simulink model "inprogress"  (R2017b)
settings: Solver=FixedStepAuto  StartTime=0.0  StopTime=10000  RelTol=1e-3  EnableMultiTasking=on
libraries: vexarmcortexlib x23
settings Model: ExtModeTrigDuration=25  Creator=Walt  LastModifiedBy=Walt
settings OptimizationCC: PassReuseOutputArgsAs=Individual arguments  MaxStackSize=64
settings DebuggingCC: ParameterTunabilityLossMsg=error
settings HardwareCC: ProdBitPerPointer=32  ProdBitPerSizeT=32  ProdBitPerPtrDiffT=32  ProdLargestAtomicInteger=Long  ProdLargestAtomicFloat=Double  ProdWordSize=32  ProdHWDeviceType=ARM Compatible->ARM Cortex
settings SFSimCC: MATLABDynamicMemAlloc=off
settings RTWCC: SystemTargetFile=ert.tlc  HardwareBoard=ARM Cortex-based VEX Microcontroller  TemplateMakefile=ert_default_tmf  GenerateReport=on  Toolchain=GNU Tools for VEX ARM Cortex  IncludeHyperlinkInReport=on  LaunchReport=on  GenerateTraceInfo=on  GenerateTraceReport=on  GenerateTraceReportSl=on  GenerateTraceReportSf=on  GenerateTraceReportEml=on
settings CodeAppCC: ForceParamTrailComments=on  IgnoreCustomStorageClasses=off  OperatorAnnotations=on  SimulinkDataObjDesc=on  SFDataObjDesc=on  InsertBlockDesc=on

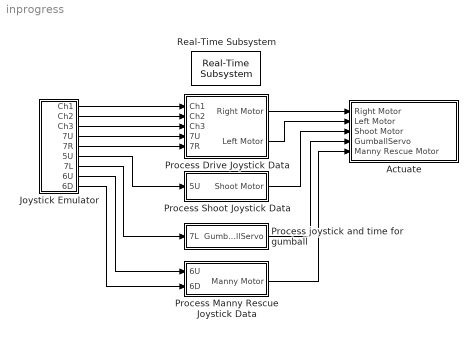
== system inprogress ==
  Actuate : Subsystem
  Joystick Emulator : Subsystem
  Process Drive Joystick Data : Subsystem
  Process Manny Rescue Joystick Data : Subsystem
  Process Shoot Joystick Data : Subsystem
  Process joystick and time for gumball : Subsystem
  Real-Time Subsystem : vexarmcortexlib/Utilities/Real-Time Subsystem  x=1
      settings: SourceProductName=Simulink Coder Support Package for ARM Cortex-based VEX Microcontroller  SourceProductBaseCode=EC_VEX_MICRO
  wires:
  Joystick Emulator/1(Ch1) -> Process Drive Joystick Data/1(Ch1)
  Joystick Emulator/2(Ch2) -> Process Drive Joystick Data/2(Ch2)
  Joystick Emulator/3(Ch3) -> Process Drive Joystick Data/3(Ch3)
  Joystick Emulator/5(7R) -> Process Drive Joystick Data/5(7R)
  Process Drive Joystick Data/1(Right Motor) -> Actuate/1(Right Motor)
  Process Drive Joystick Data/2(Left Motor) -> Actuate/2(Left Motor)
  Joystick Emulator/4(7U) -> Process Drive Joystick Data/4(7U)
  Joystick Emulator/6(5U) -> Process Shoot Joystick Data/1(5U)
  Process Shoot Joystick Data/1(Shoot Motor) -> Actuate/3(Shoot Motor)
  Joystick Emulator/8(6U) -> Process Manny Rescue Joystick Data/1(6U)
  Joystick Emulator/9(6D) -> Process Manny Rescue Joystick Data/2(6D)
  Process Manny Rescue Joystick Data/1(Manny Motor) -> Actuate/5(Manny Rescue Motor)
  Joystick Emulator/7(7L) -> Process joystick and time for gumball/1(7L)
  Process joystick and time for gumball/1(GumballServo) -> Actuate/4(GumballServo)

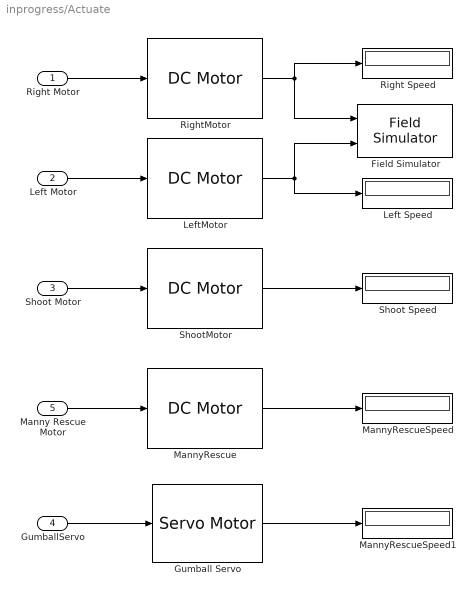
== system inprogress/Actuate ==
  Right Motor : Inport
  Left Motor : Inport  Port=2
  Shoot Motor : Inport  Port=3
  GumballServo : Inport  Port=4
  Manny Rescue Motor : Inport  Port=5
  Field Simulator : vexarmcortexlib/Utilities/Field Simulator  radius=4  space=8  range=200
      settings: SourceProductName=Simulink Coder Support Package for ARM Cortex-based VEX Microcontroller  SourceProductBaseCode=EC_VEX_MICRO
  Gumball Servo : vexarmcortexlib/Actuators/Servo Motor  motor=1  scaleFactor=60/127  SimulationOut=on
      settings: SourceProductName=Simulink Coder Support Package for ARM Cortex-based VEX Microcontroller  SourceProductBaseCode=EC_VEX_MICRO
  Left Speed : Display
  LeftMotor : vexarmcortexlib/Actuators/DC Motor  motor=2  scaleFactor=1/13.5  SimulationOut=on
      settings: SourceProductName=Simulink Coder Support Package for ARM Cortex-based VEX Microcontroller  SourceProductBaseCode=EC_VEX_MICRO
  MannyRescue : vexarmcortexlib/Actuators/DC Motor  motor=8  scaleFactor=1/13.5  SimulationOut=on
      settings: SourceProductName=Simulink Coder Support Package for ARM Cortex-based VEX Microcontroller  SourceProductBaseCode=EC_VEX_MICRO
  MannyRescueSpeed : Display
  MannyRescueSpeed1 : Display
  Right Speed : Display
  RightMotor : vexarmcortexlib/Actuators/DC Motor  motor=9  scaleFactor=1/13.5  SimulationOut=on
      settings: SourceProductName=Simulink Coder Support Package for ARM Cortex-based VEX Microcontroller  SourceProductBaseCode=EC_VEX_MICRO
  Shoot Speed : Display
  ShootMotor : vexarmcortexlib/Actuators/DC Motor  motor=3  scaleFactor=1/13.5  SimulationOut=on
      settings: SourceProductName=Simulink Coder Support Package for ARM Cortex-based VEX Microcontroller  SourceProductBaseCode=EC_VEX_MICRO
  wires:
  Shoot Motor/1 -> ShootMotor/1
  Manny Rescue Motor/1 -> MannyRescue/1
  Right Motor/1 -> RightMotor/1
  Left Motor/1 -> LeftMotor/1
  GumballServo/1 -> Gumball Servo/1
  RightMotor/1 -> Right Speed/1, Field Simulator/1
  LeftMotor/1 -> Field Simulator/2, Left Speed/1
  ShootMotor/1 -> Shoot Speed/1
  MannyRescue/1 -> MannyRescueSpeed/1
  Gumball Servo/1 -> MannyRescueSpeed1/1

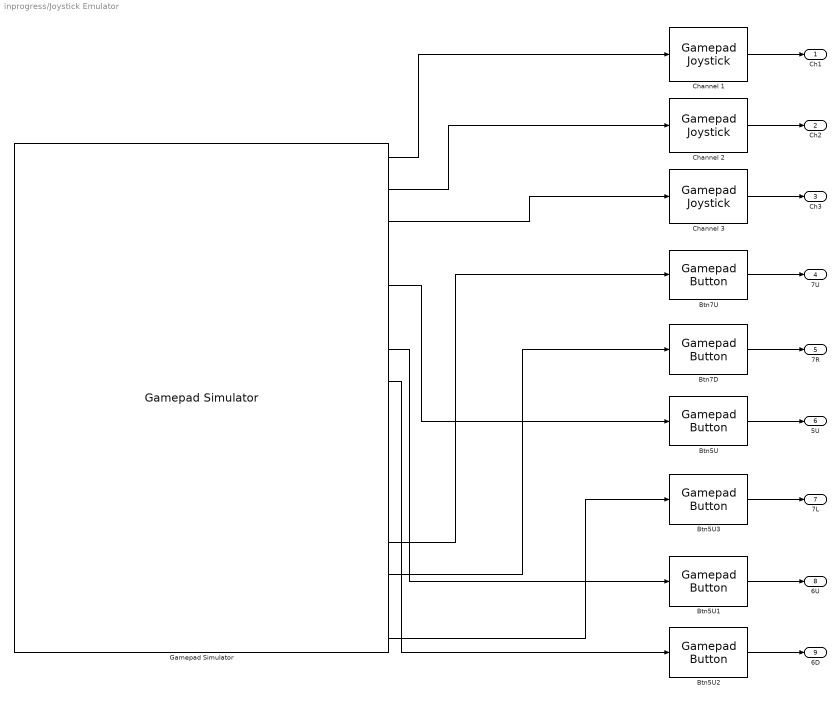
== system inprogress/Joystick Emulator ==
  Btn5U : vexarmcortexlib/Gamepad/Gamepad Button  joystick=1  chan=5  button56=Up  button78=Down  SimulationIn=on  SampleTime=0.2
      settings: SourceProductName=Simulink Coder Support Package for ARM Cortex-based VEX Microcontroller  SourceProductBaseCode=EC_VEX_MICRO
  Btn5U1 : vexarmcortexlib/Gamepad/Gamepad Button  joystick=1  chan=6  button56=Up  button78=Down  SimulationIn=on  SampleTime=0.2
      settings: SourceProductName=Simulink Coder Support Package for ARM Cortex-based VEX Microcontroller  SourceProductBaseCode=EC_VEX_MICRO
  Btn5U2 : vexarmcortexlib/Gamepad/Gamepad Button  joystick=1  chan=6  button56=Down  button78=Down  SimulationIn=on  SampleTime=0.2
      settings: SourceProductName=Simulink Coder Support Package for ARM Cortex-based VEX Microcontroller  SourceProductBaseCode=EC_VEX_MICRO
  Btn5U3 : vexarmcortexlib/Gamepad/Gamepad Button  joystick=1  chan=7  button56=Down  button78=Left  SimulationIn=on  SampleTime=0.2
      settings: SourceProductName=Simulink Coder Support Package for ARM Cortex-based VEX Microcontroller  SourceProductBaseCode=EC_VEX_MICRO
  Btn7D : vexarmcortexlib/Gamepad/Gamepad Button  joystick=1  chan=7  button56=Down  button78=Right  SimulationIn=on  SampleTime=0.2
      settings: SourceProductName=Simulink Coder Support Package for ARM Cortex-based VEX Microcontroller  SourceProductBaseCode=EC_VEX_MICRO
  Btn7U : vexarmcortexlib/Gamepad/Gamepad Button  joystick=1  chan=7  button56=Down  button78=Up  SimulationIn=on  SampleTime=0.2
      settings: SourceProductName=Simulink Coder Support Package for ARM Cortex-based VEX Microcontroller  SourceProductBaseCode=EC_VEX_MICRO
  Channel 1 : vexarmcortexlib/Gamepad/Gamepad Joystick  joystick=1  chan=1  SimulationIn=on  SampleTime=0.2
      settings: SourceProductName=Simulink Coder Support Package for ARM Cortex-based VEX Microcontroller  SourceProductBaseCode=EC_VEX_MICRO
  Channel 2 : vexarmcortexlib/Gamepad/Gamepad Joystick  joystick=1  chan=2  SimulationIn=on  SampleTime=0.2
      settings: SourceProductName=Simulink Coder Support Package for ARM Cortex-based VEX Microcontroller  SourceProductBaseCode=EC_VEX_MICRO
  Channel 3 : vexarmcortexlib/Gamepad/Gamepad Joystick  joystick=1  chan=3  SimulationIn=on  SampleTime=0.2
      settings: SourceProductName=Simulink Coder Support Package for ARM Cortex-based VEX Microcontroller  SourceProductBaseCode=EC_VEX_MICRO
  Gamepad Simulator : vexarmcortexlib/Utilities/Gamepad Simulator  WhichPad=Logitech Gamepad  JoyId=1
      settings: SourceProductName=Simulink Coder Support Package for ARM Cortex-based VEX Microcontroller  SourceProductBaseCode=EC_VEX_MICRO
  Ch1 : Outport
  Ch2 : Outport  Port=2
  Ch3 : Outport  Port=3
  7U : Outport  Port=4
  7R : Outport  Port=5
  5U : Outport  Port=6
  7L : Outport  Port=7
  6U : Outport  Port=8
  6D : Outport  Port=9
  wires:
  Gamepad Simulator/3 -> Channel 3/1
  Channel 3/1 -> Ch3/1
  Gamepad Simulator/14 -> Btn7D/1
  Gamepad Simulator/2 -> Channel 2/1
  Channel 2/1 -> Ch2/1
  Channel 1/1 -> Ch1/1
  Gamepad Simulator/1 -> Channel 1/1
  Btn7D/1 -> 7R/1
  Gamepad Simulator/13 -> Btn7U/1
  Btn7U/1 -> 7U/1
  Gamepad Simulator/5 -> Btn5U/1
  Btn5U/1 -> 5U/1
  Gamepad Simulator/7 -> Btn5U1/1
  Gamepad Simulator/8 -> Btn5U2/1
  Btn5U2/1 -> 6D/1
  Btn5U1/1 -> 6U/1
  Btn5U3/1 -> 7L/1
  Gamepad Simulator/16 -> Btn5U3/1

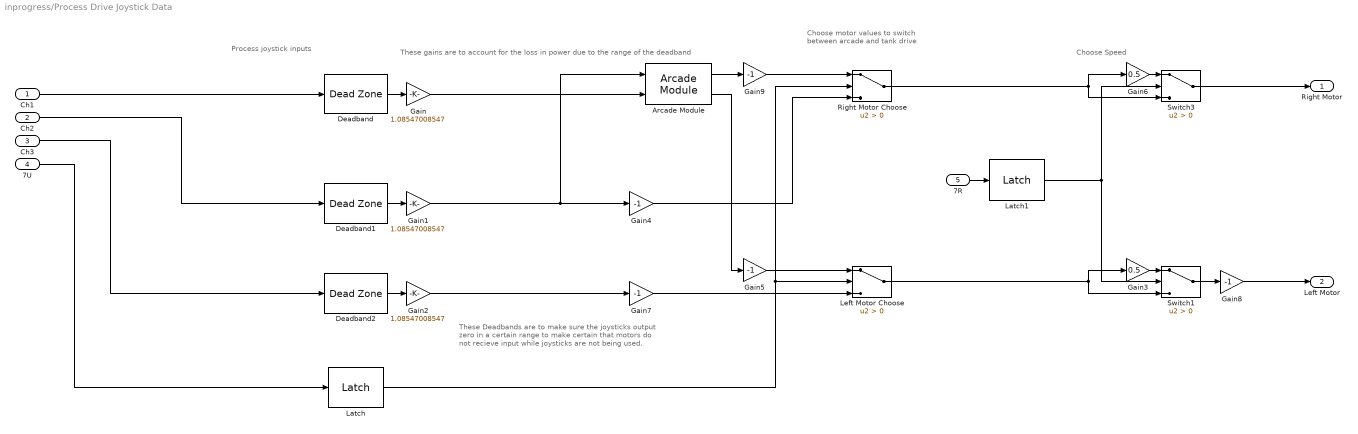
== system inprogress/Process Drive Joystick Data ==
  note: Choose Speed
  note: Process joystick inputs
  note: Choose motor values to
      | switch between arcade
      | and tank drive
  note: These Deadbands are to make sure the joysticks output zero in a certain range to make certain that motors do not recieve input while joysticks are not being used.
  note: These gains are to account for the loss in power due to the range of the deadband
  Ch1 : Inport
  Ch2 : Inport  Port=2
  Ch3 : Inport  Port=3
  7U : Inport  Port=4
  7R : Inport  Port=5
  Arcade Module : vexarmcortexlib/Utilities/Arcade Module
      settings: SourceProductName=Simulink Coder Support Package for ARM Cortex-based VEX Microcontroller  SourceProductBaseCode=EC_VEX_MICRO
  Deadband : DeadZone  LowerValue=-10  UpperValue=10  SaturateOnIntegerOverflow=on
  Deadband1 : DeadZone  LowerValue=-10  UpperValue=10  SaturateOnIntegerOverflow=on
  Deadband2 : DeadZone  LowerValue=-10  UpperValue=10  SaturateOnIntegerOverflow=on
  Gain : Gain  Gain=1.08547008547
  Gain1 : Gain  Gain=1.08547008547
  Gain2 : Gain  Gain=1.08547008547
  Gain3 : Gain  Gain=0.5
  Gain{4..5,7..9} (5 alike) : Gain  Gain=-1
  Gain6 : Gain  Gain=0.5
  Latch : vexarmcortexlib/Utilities/Latch  output0=off
      settings: SourceProductName=Simulink Coder Support Package for ARM Cortex-based VEX Microcontroller  SourceProductBaseCode=EC_VEX_MICRO
  Latch1 : vexarmcortexlib/Utilities/Latch  output0=off
      settings: SourceProductName=Simulink Coder Support Package for ARM Cortex-based VEX Microcontroller  SourceProductBaseCode=EC_VEX_MICRO
  Left Motor Choose : Switch  Criteria=u2 > Threshold
  Right Motor Choose : Switch  Criteria=u2 > Threshold
  Switch1 : Switch  Criteria=u2 > Threshold
  Switch3 : Switch  Criteria=u2 > Threshold
  Right Motor : Outport
  Left Motor : Outport  Port=2
  wires:
  Arcade Module/1 -> Gain9/1
  7R/1 -> Latch1/1
  Gain2/1 -> Gain7/1
  Gain3/1 -> Switch1/1
  Left Motor Choose/1 -> Switch1/3, Gain3/1
  Arcade Module/2 -> Gain5/1
  Deadband/1 -> Gain/1
  Deadband1/1 -> Gain1/1
  Deadband2/1 -> Gain2/1
  Right Motor Choose/1 -> Gain6/1, Switch3/3
  Gain6/1 -> Switch3/1
  Latch/1 -> Left Motor Choose/2, Right Motor Choose/2
  Gain1/1 -> Gain4/1, Arcade Module/1
  Gain/1 -> Arcade Module/2
  Ch1/1 -> Deadband/1
  Ch2/1 -> Deadband1/1
  7U/1 -> Latch/1
  Ch3/1 -> Deadband2/1
  Gain4/1 -> Right Motor Choose/3
  Gain7/1 -> Left Motor Choose/3
  Switch1/1 -> Gain8/1
  Switch3/1 -> Right Motor/1
  Gain8/1 -> Left Motor/1
  Gain5/1 -> Left Motor Choose/1
  Gain9/1 -> Right Motor Choose/1
  Latch1/1 -> Switch3/2, Switch1/2

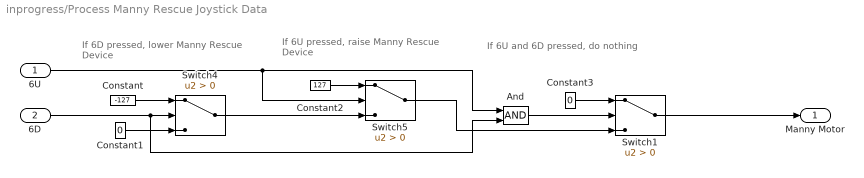
== system inprogress/Process Manny Rescue Joystick Data ==
  note: If 6U and 6D pressed,
      | do nothing
  note: If 6U pressed, raise
      | Manny Rescue Device
  note: If 6D pressed, lower Manny
      | Rescue Device
  6U : Inport
  6D : Inport  Port=2
  And : Logic  IconShape=distinctive  AllPortsSameDT=off  OutDataTypeStr=boolean
  Constant : Constant  Value=-127
  Constant1 : Constant  Value=0
  Constant2 : Constant  Value=127
  Constant3 : Constant  Value=0
  Switch1 : Switch  Criteria=u2 > Threshold
  Switch4 : Switch  Criteria=u2 > Threshold
  Switch5 : Switch  Criteria=u2 > Threshold
  Manny Motor : Outport
  wires:
  Constant/1 -> Switch4/1
  Constant1/1 -> Switch4/3
  Switch4/1 -> Switch5/3
  Constant2/1 -> Switch5/1
  6U/1 -> Switch5/2, And/1
  6D/1 -> And/2, Switch4/2
  Switch1/1 -> Manny Motor/1
  Switch5/1 -> Switch1/3
  And/1 -> Switch1/2
  Constant3/1 -> Switch1/1

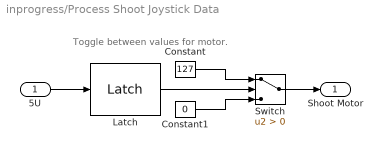
== system inprogress/Process Shoot Joystick Data ==
  note: Toggle between values for motor.
  5U : Inport
  Constant : Constant  Value=127
  Constant1 : Constant  Value=0
  Latch : vexarmcortexlib/Utilities/Latch  output0=off
      settings: SourceProductName=Simulink Coder Support Package for ARM Cortex-based VEX Microcontroller  SourceProductBaseCode=EC_VEX_MICRO
  Switch : Switch  Criteria=u2 > Threshold
  Shoot Motor : Outport
  wires:
  Switch/1 -> Shoot Motor/1
  Constant/1 -> Switch/1
  Constant1/1 -> Switch/3
  5U/1 -> Latch/1
  Latch/1 -> Switch/2

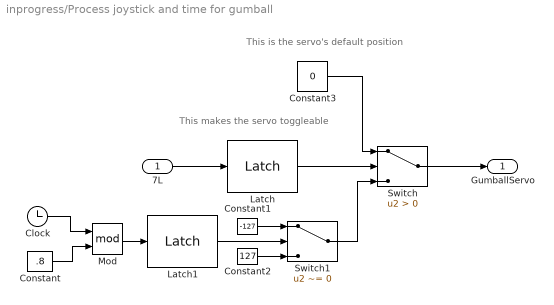
== system inprogress/Process joystick and time for gumball ==
  note: This makes the servo toggleable
  note: This is the servo's default position
  7L : Inport
  Clock : Clock
  Constant : Constant  Value=.8
  Constant1 : Constant  Value=-127
  Constant2 : Constant  Value=127
  Constant3 : Constant  Value=0
  Latch : vexarmcortexlib/Utilities/Latch  output0=off
      settings: SourceProductName=Simulink Coder Support Package for ARM Cortex-based VEX Microcontroller  SourceProductBaseCode=EC_VEX_MICRO
  Latch1 : vexarmcortexlib/Utilities/Latch  output0=off
      settings: SourceProductName=Simulink Coder Support Package for ARM Cortex-based VEX Microcontroller  SourceProductBaseCode=EC_VEX_MICRO
  Mod : Math  Operator=mod  SaturateOnIntegerOverflow=on
  Switch : Switch  Criteria=u2 > Threshold
  Switch1 : Switch  Criteria=u2 ~= 0
  GumballServo : Outport
  wires:
  Constant3/1 -> Switch/1
  Latch/1 -> Switch/2
  Switch/1 -> GumballServo/1
  7L/1 -> Latch/1
  Clock/1 -> Mod/1
  Constant/1 -> Mod/2
  Mod/1 -> Latch1/1
  Latch1/1 -> Switch1/2
  Constant1/1 -> Switch1/1
  Constant2/1 -> Switch1/3
  Switch1/1 -> Switch/3
